simulink model "ARDC_IPMSM_Control"  (R2021b)
settings: Solver=VariableStepAuto  StartTime=0.0  StopTime=10  FixedStep=1e-6  MaxStep=1e-6  RelTol=1e-3
values from neighbouring files (symbols this model uses):
  B = 4.924e-4    (= 0.0004924)    [ARDC_PMSMControl_TreadmillLoad.m]
  J = 0.002700    (= 0.0027)    [ARDC_PMSMControl_TreadmillLoad.m]
  Kinv = Vdc/sqrt(2)    [ARDC_PMSMControl_TreadmillLoad.m]
  L_Stride = 1.8    [ARDC_PMSMControl_TreadmillLoad.m]
  Ld = 3.752e-4    (= 0.0003752)    [ARDC_PMSMControl_TreadmillLoad.m]
  Lq = 4.148e-4    (= 0.0004148)    [ARDC_PMSMControl_TreadmillLoad.m]
  P = 4    [ARDC_PMSMControl_TreadmillLoad.m]
  psim = 0.1194    [ARDC_PMSMControl_TreadmillLoad.m]
  R_roller = 0.1    [ARDC_PMSMControl_TreadmillLoad.m]
  Rs = 0.02    [ARDC_PMSMControl_TreadmillLoad.m]
  TreadMill_Enable = 1    [ARDC_PMSMControl_TreadmillLoad.m]
  Ts = 25e-6    (= 2.5e-05)    [ARDC_PMSMControl_TreadmillLoad.m]
  Tsw = 1/Fsw    (= 5e-05)    [ARDC_PMSMControl_TreadmillLoad.m]
  Vdc = 200    [ARDC_PMSMControl_TreadmillLoad.m]
undefined symbols (not defined in the file or in its folder): DiscIntNeverNeededParam
libraries: spsMosfetLib x6, slpidlib x3, spsVoltageMeasurementLib x3, simulink x2, spsPermanentMagnetSynchronousMachineLib x1, spsDCVoltageSourceLib x1, spsFirstOrderFilterLib x1, spspowerguiLib x1, spsTriangleGeneratorLib x1
settings Model: Creator=desai  LastModifiedBy=desai
settings DebuggingCC: UnderSpecifiedDimensionMsg=warning

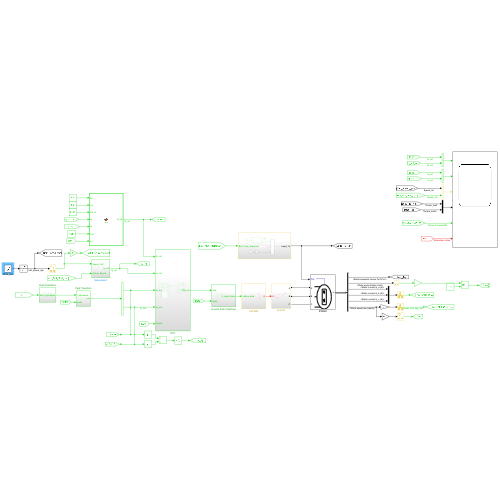
[thumbnail: Simulink's stored preview of the top-level diagram]
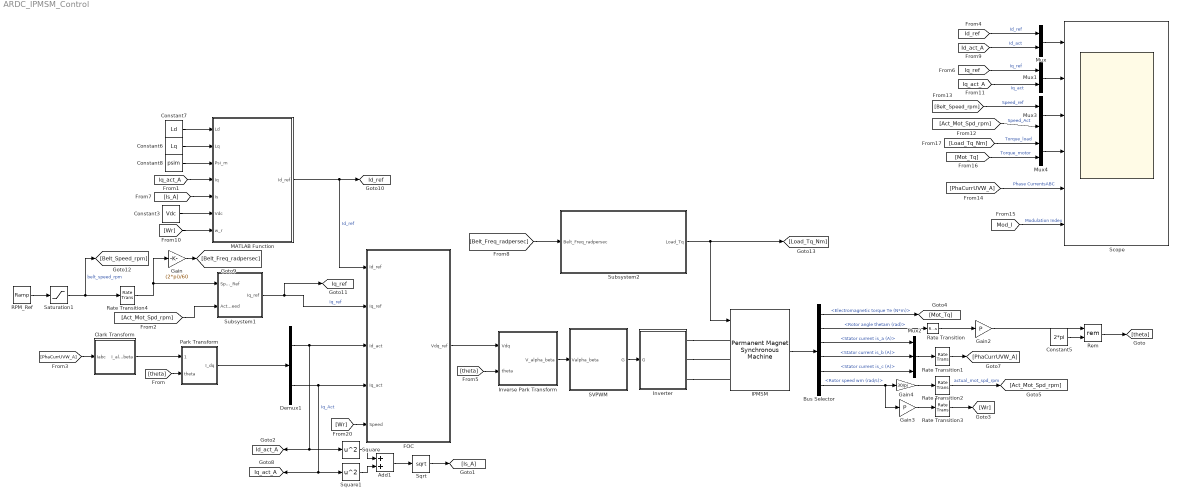
== system ARDC_IPMSM_Control ==
  Add1 : Sum
  Bus Selector : BusSelector  OutputSignals=Electromagnetic torque Te (N*m),Rotor angle thetam (rad),Stator current is_a (A),Stator current is_b (A),Stator current is_c (A),Rotor speed wm (rad/s)
  Clark Transform : Subsystem
  Constant3 : Constant  Value=Vdc  SampleTime=Ts
  Constant5 : Constant  Value=2*pi  SampleTime=Ts
  Constant6 : Constant  Value=Lq  SampleTime=Ts
  Constant7 : Constant  Value=Ld  SampleTime=Ts
  Constant8 : Constant  Value=psim  SampleTime=Ts
  Demux1 : Demux  Outputs=2
  FOC : Subsystem
  Gain : Gain  Gain=(2*pi)/60
  Gain2 : Gain  Gain=P
  Gain3 : Gain  Gain=P
  Gain4 : Gain  Gain=30/pi
  IPMSM : spsPermanentMagnetSynchronousMachineLib/Permanent Magnet Synchronous Machine  NbPhases=3  FluxDistribution=Sinusoidal  RotorType=Salient-pole  MechanicalLoad=Torque Tm  PresetModel=No  ShowDetailedParameters=on  MeasurementBus=off  Resistance=Rs  Inductance=8.5e-3  dqInductances=[Ld Lq]  La=0.000395  MachineConstant=Flux linkage established by magnets (V.s)  Flux=psim  VoltageCst=86.6271  TorqueCst=0.7164  Flat=120  Mechanical=[J B P 0]  PolePairs=P  InitialConditions=[0,0, 0,0]  InitialConditions5ph=[0 0 0 0 0 0]  RefAngle=Aligned with phase A axis (original Park)  IterativeDiscreteModel=Trapezoidal non iterative  TsBlock=-1  TsPowergui=0
  Inverse Park Transform : Subsystem
  Inverter : Subsystem
  MATLAB Function : MATLAB Function  TreatAsAtomicUnit=on
  Mux{,1,3..4} (4 alike) : Mux  Inputs=2
  Mux2 : Mux  Inputs=3
  Park Transform : Subsystem
  RPM_Ref : simulink/Sources/Ramp  slope=240  start=0  InitialOutput=0
  Rate Transition{,1..4} (5 alike) : RateTransition  OutPortSampleTime=Ts
  Rem : Math  Operator=rem  SaturateOnIntegerOverflow=on
  SVPWM : Subsystem
  Saturation1 : Saturate  UpperLimit=1200  LowerLimit=0
  Scope : Scope  NumInputPorts=6
  Sqrt : Sqrt  SaturateOnIntegerOverflow=on
  Square : Math  Operator=square  SaturateOnIntegerOverflow=on
  Square1 : Math  Operator=square  SaturateOnIntegerOverflow=on
  Subsystem1 : Subsystem
  Subsystem2 : Subsystem
  tag scope: Id_act_A=global, Id_ref=global, Iq_act_A=global, Iq_ref=global
  wires:
  IPMSM/1 -> Bus Selector/1
  Bus Selector/2 -> Rate Transition/1  "<Rotor angle thetam (rad)>"
  Mux2/1 -> Rate Transition1/1
  Clark Transform/1(I_alphabeta) -> Park Transform/1(I_alphabeta)
  SVPWM/1(G) -> Inverter/1(G)
  [Wr] -> FOC/5(Speed)
  FOC/1(Vdq_ref) -> Inverse Park Transform/1(Vdq)
  Demux1/2 -> [Iq_act_A], Square1/1, FOC/4(Iq_act)  "Iq_Act"
  Demux1/1 -> [Id_act_A], Square/1, FOC/3(Id_act)
  [theta] -> Inverse Park Transform/2(theta)
  Inverse Park Transform/1(V_alpha_beta) -> SVPWM/1(Valpha_beta)
  [theta] -> Park Transform/2(theta)
  Rate Transition/1 -> Gain2/1
  Constant5/1 -> Rem/2
  Rem/1 -> [theta]
  Gain3/1 -> Rate Transition3/1
  Bus Selector/1 -> [Mot_Tq]  "<Electromagnetic torque Te (N*m)>"
  [PhaCurrUVW_A] -> Clark Transform/1(Iabc)
  Gain4/1 -> Rate Transition2/1
  Add1/1 -> Sqrt/1
  Square/1 -> Add1/1
  Square1/1 -> Add1/2
  Sqrt/1 -> [Is_A]
  [Is_A] -> MATLAB Function/5(Is)
  [Iq_act_A] -> MATLAB Function/4(Iq)
  Constant3/1 -> MATLAB Function/6(Vdc)
  [Wr] -> MATLAB Function/7(w_r)
  Constant6/1 -> MATLAB Function/2(Lq)
  Constant7/1 -> MATLAB Function/1(Ld)
  Constant8/1 -> MATLAB Function/3(Psi_m)
  MATLAB Function/1(Id_ref) -> [Id_ref], FOC/1(Id_ref)  "Id_ref"
  RPM_Ref/1 -> Saturation1/1
  Saturation1/1 -> [Belt_Speed_rpm], Rate Transition4/1  "belt_speed_rpm"
  Rate Transition4/1 -> Gain/1, Subsystem1/1(Speed_Ref)
  [Act_Mot_Spd_rpm] -> Subsystem1/2(Actual_Speed)
  Gain/1 -> [Belt_Freq_radpersec]
  Bus Selector/3 -> Mux2/1  "<Stator current is_a (A)>"
  Bus Selector/4 -> Mux2/2  "<Stator current is_b (A)>"
  Bus Selector/5 -> Mux2/3  "<Stator current is_c (A)>"
  Bus Selector/6 -> Gain3/1, Gain4/1  "<Rotor speed wm (rad/s)>"
  Rate Transition3/1 -> [Wr]
  Gain2/1 -> Rem/1
  Subsystem1/1(Iq_ref) -> [Iq_ref], FOC/2(Iq_ref)  "Iq_ref"
  Rate Transition2/1 -> [Act_Mot_Spd_rpm]  "actual_mot_spd_rpm"
  Park Transform/1(I_dq) -> Demux1/1
  Rate Transition1/1 -> [PhaCurrUVW_A]
  [Id_ref] -> Mux/1  "Id_ref"
  [Id_act_A] -> Mux/2  "Id_act"
  [Iq_act_A] -> Mux1/2  "Iq_act"
  [Iq_ref] -> Mux1/1  "Iq_ref"
  [Belt_Speed_rpm] -> Mux3/1  "Speed_ref"
  [Act_Mot_Spd_rpm] -> Mux3/2  "Speed_Act"
  Mux/1 -> Scope/1
  Mux1/1 -> Scope/2
  Mux3/1 -> Scope/3
  [PhaCurrUVW_A] -> Scope/5  "Phase CurrentsABC"
  [Mod_I] -> Scope/6  "Modulation Index"
  [Mot_Tq] -> Mux4/2  "Torque_motor"
  [Load_Tq_Nm] -> Mux4/1  "Torque_load"
  Mux4/1 -> Scope/4
  [Belt_Freq_radpersec] -> Subsystem2/1(Belt_Freq_radpersec)
  Subsystem2/1(Load_Tq) -> IPMSM/1, [Load_Tq_Nm]
  connections:
  Inverter/RConn1 -- IPMSM/LConn1
  Inverter/RConn2 -- IPMSM/LConn2
  Inverter/RConn3 -- IPMSM/LConn3

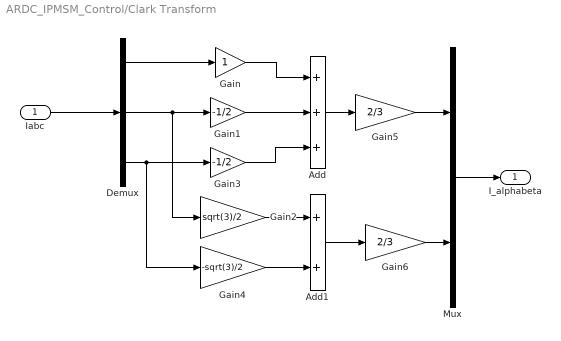
== system ARDC_IPMSM_Control/Clark Transform ==
  Iabc : Inport
  Add : Sum  Inputs=+++
  Add1 : Sum
  Demux : Demux  Outputs=3
  Gain : Gain
  Gain1 : Gain  Gain=-1/2
  Gain2 : Gain  Gain=sqrt(3)/2
  Gain3 : Gain  Gain=-1/2
  Gain4 : Gain  Gain=-sqrt(3)/2
  Gain5 : Gain  Gain=2/3
  Gain6 : Gain  Gain=2/3
  Mux : Mux  Inputs=2
  I_alphabeta : Outport  VectorParamsAs1DForOutWhenUnconnected=off
  wires:
  Gain/1 -> Add/1
  Demux/2 -> Gain1/1, Gain2/1
  Demux/3 -> Gain3/1, Gain4/1
  Gain1/1 -> Add/2
  Gain3/1 -> Add/3
  Gain4/1 -> Add1/2
  Gain2/1 -> Add1/1
  Demux/1 -> Gain/1
  Iabc/1 -> Demux/1
  Mux/1 -> I_alphabeta/1
  Add/1 -> Gain5/1
  Add1/1 -> Gain6/1
  Gain5/1 -> Mux/1
  Gain6/1 -> Mux/2

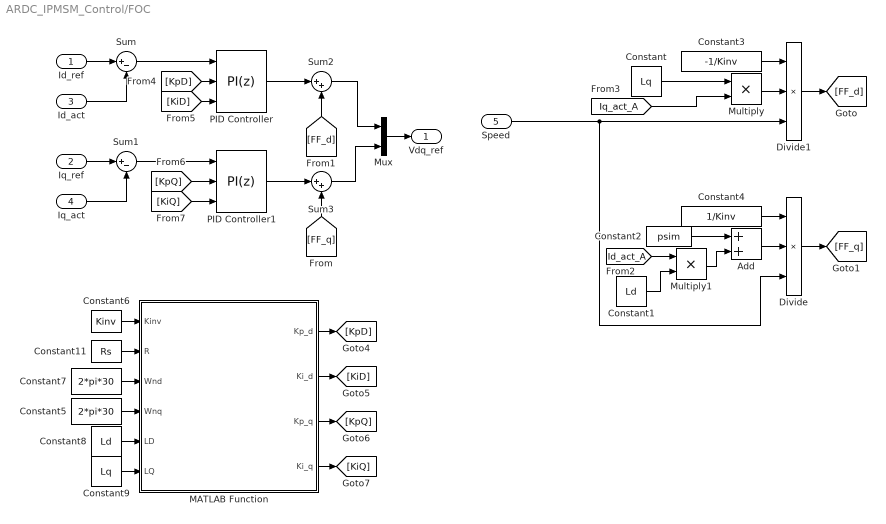
== system ARDC_IPMSM_Control/FOC ==
  Id_ref : Inport
  Iq_ref : Inport  Port=2
  Id_act : Inport  Port=3
  Iq_act : Inport  Port=4
  Speed : Inport  Port=5
  Add : Sum
  Constant : Constant  Value=Lq  SampleTime=Ts
  Constant1 : Constant  Value=Ld  SampleTime=Ts
  Constant11 : Constant  Value=Rs  SampleTime=Ts
  Constant2 : Constant  Value=psim  SampleTime=Ts
  Constant3 : Constant  Value=-1/Kinv  SampleTime=Ts
  Constant4 : Constant  Value=1/Kinv  SampleTime=Ts
  Constant5 : Constant  Value=2*pi*30  SampleTime=Ts
  Constant6 : Constant  Value=Kinv  SampleTime=Ts
  Constant7 : Constant  Value=2*pi*30  SampleTime=Ts
  Constant8 : Constant  Value=Ld  SampleTime=Ts
  Constant9 : Constant  Value=Lq  SampleTime=Ts
  Divide : Product  Inputs=***
  Divide1 : Product  Inputs=***
  MATLAB Function : MATLAB Function  TreatAsAtomicUnit=on
  Multiply : Product
  Multiply1 : Product
  Mux : Mux  Inputs=2
  PID Controller : slpidlib/PID Controller  Controller=PI  Form=Parallel  TimeDomain=Discrete-time  UseExternalTs=off  SampleTime=Ts  IntegratorMethod=Forward Euler  FilterMethod=Forward Euler  ControllerParametersSource=external  P=(2*1000*Ld - Rs)/Kinv  I=(Ld*2*1000*1000)/Kinv  D=0  UseFilter=on  N=100  TunerSelectOption=Transfer Function Based (PID Tuner App)  InitialConditionSource=internal  InitialConditionForIntegrator=0  InitialConditionForFilter=0  DifferentiatorICPrevScaledInput=0  ExternalReset=none  IgnoreLimit=on  TrackingMode=off  Kt=1  LimitOutput=off  SatLimitsSource=internal  UpperSaturationLimit=inf  LowerSaturationLimit=-inf  LinearizeAsGain=on  AntiWindupMode=none  Kb=1  POutMin=[]  POutMax=[]  IOutMin=[]  IOutMax=[]  DOutMin=[]  DOutMax=[]  NOutMin=[]  NOutMax=[]  SumOutMin=[]  SumOutMax=[]  SaturationOutMin=[]  SaturationOutMax=[]  PParamMin=[]  PParamMax=[]  IParamMin=[]  IParamMax=[]  DParamMin=[]  DParamMax=[]  NParamMin=[]  NParamMax=[]  KbParamMin=[]  KbParamMax=[]  KtParamMin=[]  KtParamMax=[]  KbOutMin=[]  KbOutMax=[]  KtOutMin=[]  KtOutMax=[]  IntegratorOutMin=[]  IntegratorOutMax=[]  FilterOutMin=[]  FilterOutMax=[]  SumI1OutMin=[]  SumI1OutMax=[]  SumI2OutMin=[]  SumI2OutMax=[]  SumI3OutMin=[]  SumI3OutMax=[]  SumI4OutMin=[]  SumI4OutMax=[]  SumDOutMin=[]  SumDOutMax=[]  DifferentiatorOutMin=[]  DifferentiatorOutMax=[]  FilterDiffOutCoefMin=[]  FilterDiffOutCoefMax=[]  ReciprocalOutMin=[]  ReciprocalOutMax=[]  SumDenOutMin=[]  SumDenOutMax=[]  SumNumOutMin=[]  SumNumOutMax=[]  DivideOutMin=[]  DivideOutMax=[]  UdiffTsProdOutMin=[]  UdiffTsProdOutMax=[]  NTsProdOutMin=[]  NTsProdOutMax=[]  UintegralTsProdOutMin=[]  UintegralTsProdOutMax=[]  UngainTsProdOutMin=[]  UngainTsProdOutMax=[]  IntegratorContinuousStateAttributes=''  IntegratorStateMustResolveToSignalObject=off  IntegratorRTWStateStorageClass=Auto  FilterContinuousStateAttributes=''  FilterStateMustResolveToSignalObject=off  FilterRTWStateStorageClass=Auto  ParallelPVariant=ExternalParameters  IdealPVariant=Disabled  IVariant=ExternalParameters  DVariant=Disabled  IntegratorVariant=Discrete  SatVariant=Disabled  AWVariant=Passthrough  PCopyVariant=Disabled  TRVariant=Disabled  FdbkBlocksVariant=Forward  IdealPFdbkVariant=Disabled  SatFdbkVariant=Disabled  DerivativeFilterVariant=Disabled  NVariant=Disabled  NCopyVariant=Disabled_SignalSpec  FilterICVariant=Disabled  IntegratorICVariant=InternalICs  ExternalResetVariant=Disabled  TRSumVariant=Passthrough  SumFdbkVariant=Disabled  SumVariant=Sum_PI  TsampFilterVariant=InternalTs  TsampNgainVariant=Passthrough  TsampIntegralVariant=Passthrough  ExternalSaturationOutDataTypeStr=Inherit: Same as second input
  PID Controller1 : slpidlib/PID Controller  Controller=PI  Form=Parallel  TimeDomain=Discrete-time  UseExternalTs=off  SampleTime=Ts  IntegratorMethod=Forward Euler  FilterMethod=Forward Euler  ControllerParametersSource=external  P=(2*1000*Lq - Rs)/Kinv  I=(Lq*2*1000*1000)/Kinv  D=0  UseFilter=on  N=100  TunerSelectOption=Transfer Function Based (PID Tuner App)  InitialConditionSource=internal  InitialConditionForIntegrator=0  InitialConditionForFilter=0  DifferentiatorICPrevScaledInput=0  ExternalReset=none  TrackingMode=off  Kt=1  LimitOutput=off  SatLimitsSource=internal  UpperSaturationLimit=inf  LowerSaturationLimit=-inf  LinearizeAsGain=on  AntiWindupMode=none  Kb=1  POutMin=[]  POutMax=[]  IOutMin=[]  IOutMax=[]  DOutMin=[]  DOutMax=[]  NOutMin=[]  NOutMax=[]  SumOutMin=[]  SumOutMax=[]  SaturationOutMin=[]  SaturationOutMax=[]  PParamMin=[]  PParamMax=[]  IParamMin=[]  IParamMax=[]  DParamMin=[]  DParamMax=[]  NParamMin=[]  NParamMax=[]  KbParamMin=[]  KbParamMax=[]  KtParamMin=[]  KtParamMax=[]  KbOutMin=[]  KbOutMax=[]  KtOutMin=[]  KtOutMax=[]  IntegratorOutMin=[]  IntegratorOutMax=[]  FilterOutMin=[]  FilterOutMax=[]  SumI1OutMin=[]  SumI1OutMax=[]  SumI2OutMin=[]  SumI2OutMax=[]  SumI3OutMin=[]  SumI3OutMax=[]  SumI4OutMin=[]  SumI4OutMax=[]  SumDOutMin=[]  SumDOutMax=[]  DifferentiatorOutMin=[]  DifferentiatorOutMax=[]  FilterDiffOutCoefMin=[]  FilterDiffOutCoefMax=[]  ReciprocalOutMin=[]  ReciprocalOutMax=[]  SumDenOutMin=[]  SumDenOutMax=[]  SumNumOutMin=[]  SumNumOutMax=[]  DivideOutMin=[]  DivideOutMax=[]  UdiffTsProdOutMin=[]  UdiffTsProdOutMax=[]  NTsProdOutMin=[]  NTsProdOutMax=[]  UintegralTsProdOutMin=[]  UintegralTsProdOutMax=[]  UngainTsProdOutMin=[]  UngainTsProdOutMax=[]  IntegratorContinuousStateAttributes=''  IntegratorStateMustResolveToSignalObject=off  IntegratorRTWStateStorageClass=Auto  FilterContinuousStateAttributes=''  FilterStateMustResolveToSignalObject=off  FilterRTWStateStorageClass=Auto  ParallelPVariant=ExternalParameters  IdealPVariant=Disabled  IVariant=ExternalParameters  DVariant=Disabled  IntegratorVariant=Discrete  SatVariant=Disabled  AWVariant=Passthrough  PCopyVariant=Disabled  TRVariant=Disabled  FdbkBlocksVariant=Forward  IdealPFdbkVariant=Disabled  SatFdbkVariant=Disabled  DerivativeFilterVariant=Disabled  NVariant=Disabled  NCopyVariant=Disabled_SignalSpec  FilterICVariant=Disabled  IntegratorICVariant=InternalICs  ExternalResetVariant=Disabled  TRSumVariant=Passthrough  SumFdbkVariant=Disabled  SumVariant=Sum_PI  TsampFilterVariant=InternalTs  TsampNgainVariant=Passthrough  TsampIntegralVariant=Passthrough  ExternalSaturationOutDataTypeStr=Inherit: Same as second input
  Sum : Sum  Inputs=|+-
  Sum1 : Sum  Inputs=|+-
  Sum2 : Sum  Inputs=|++
  Sum3 : Sum  Inputs=|++
  Vdq_ref : Outport  VectorParamsAs1DForOutWhenUnconnected=off
  wires:
  Id_ref/1 -> Sum/1
  Iq_ref/1 -> Sum1/1
  Id_act/1 -> Sum/2
  Sum1/1 -> PID Controller1/1
  Sum/1 -> PID Controller/1
  PID Controller/1 -> Sum2/1
  PID Controller1/1 -> Sum3/1
  Sum2/1 -> Mux/1
  Sum3/1 -> Mux/2
  Mux/1 -> Vdq_ref/1
  Iq_act/1 -> Sum1/2
  Constant1/1 -> Multiply1/2
  Constant/1 -> Multiply/1
  Multiply/1 -> Divide1/2
  [FF_q] -> Sum3/2
  [FF_d] -> Sum2/2
  Divide/1 -> [FF_q]
  Speed/1 -> Divide/3, Divide1/3
  Multiply1/1 -> Add/2
  Constant2/1 -> Add/1
  Add/1 -> Divide/2
  [Id_act_A] -> Multiply1/1
  [Iq_act_A] -> Multiply/2
  Constant3/1 -> Divide1/1
  Divide1/1 -> [FF_d]
  Constant4/1 -> Divide/1
  Constant8/1 -> MATLAB Function/5(LD)
  Constant9/1 -> MATLAB Function/6(LQ)
  Constant7/1 -> MATLAB Function/3(Wnd)
  MATLAB Function/4(Ki_q) -> [KiQ]
  MATLAB Function/3(Kp_q) -> [KpQ]
  MATLAB Function/2(Ki_d) -> [KiD]
  MATLAB Function/1(Kp_d) -> [KpD]
  [KpD] -> PID Controller/2
  [KiD] -> PID Controller/3
  [KpQ] -> PID Controller1/2
  [KiQ] -> PID Controller1/3
  Constant6/1 -> MATLAB Function/1(Kinv)
  Constant11/1 -> MATLAB Function/2(R)
  Constant5/1 -> MATLAB Function/4(Wnq)

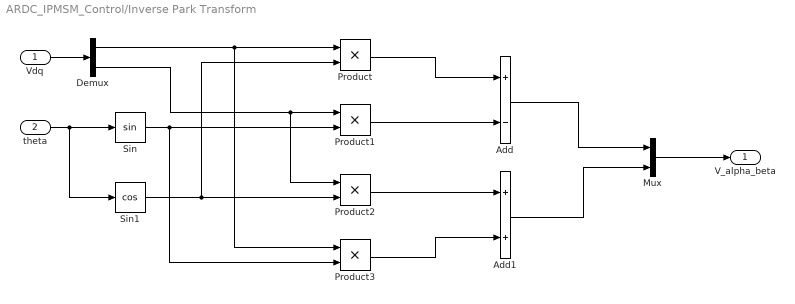
== system ARDC_IPMSM_Control/Inverse Park Transform ==
  Vdq : Inport
  theta : Inport  Port=2
  Add : Sum  Inputs=+-
  Add1 : Sum
  Demux : Demux  Outputs=2
  Mux : Mux  Inputs=2
  Product{,1..3} (4 alike) : Product
  Sin : Trigonometry
  Sin1 : Trigonometry  Operator=cos
  V_alpha_beta : Outport  VectorParamsAs1DForOutWhenUnconnected=off
  wires:
  Vdq/1 -> Demux/1
  Demux/1 -> Product/1, Product3/1
  Sin1/1 -> Product2/2, Product/2
  Product/1 -> Add/1
  Demux/2 -> Product2/1, Product1/1
  Product1/1 -> Add/2
  Sin/1 -> Product1/2, Product3/2
  Product3/1 -> Add1/2
  Product2/1 -> Add1/1
  theta/1 -> Sin/1, Sin1/1
  Add/1 -> Mux/1
  Add1/1 -> Mux/2
  Mux/1 -> V_alpha_beta/1

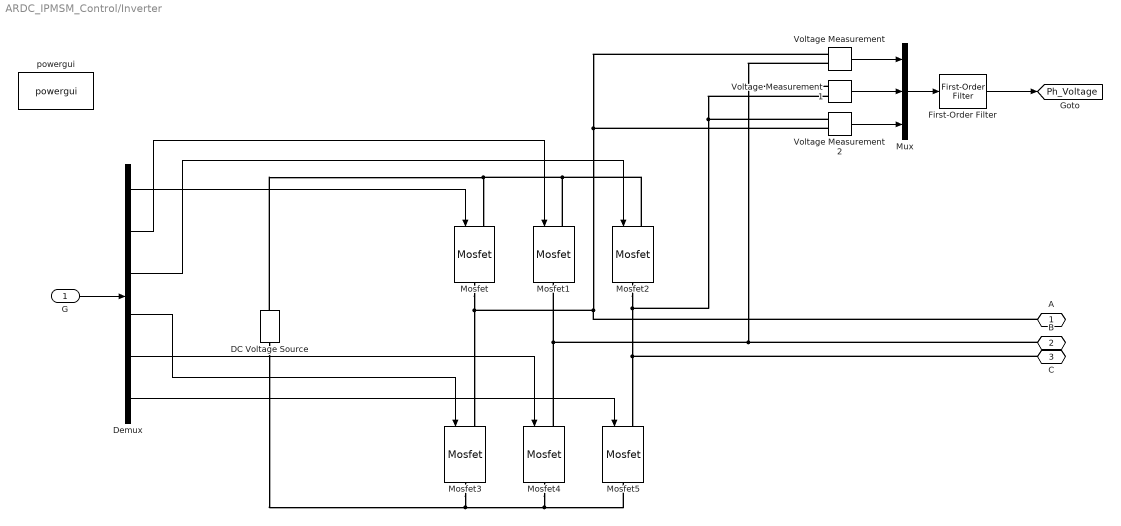
== system ARDC_IPMSM_Control/Inverter ==
  G : Inport
  DC Voltage Source : spsDCVoltageSourceLib/DC Voltage Source  Amplitude=Vdc  Measurements=None
  Demux : Demux  Outputs=6
  First-Order Filter : spsFirstOrderFilterLib/First-Order Filter  FilterType=Lowpass  Tc=1/(2*pi*200)  Ts=0  Initialize=off  Vac_Init=[0, 0, 60]  Vdc_Init=0  PlotResponse=off  FreqRange="[0,  200,  1]"
  Mosfet{,1..5} (6 alike) : spsMosfetLib/Mosfet  Ron=0.05  Lon=0  Rd=0.01  Vfd=0  IC=0  Rs=1e5  Cs=inf  Measurements=off
  Mux : Mux  Inputs=3
  Voltage Measurement : spsVoltageMeasurementLib/Voltage Measurement  PhasorSimulation=off  OutputType=Complex  PSBequivalent=0
  Voltage Measurement1 : spsVoltageMeasurementLib/Voltage Measurement  PhasorSimulation=off  OutputType=Complex  PSBequivalent=0
  Voltage Measurement2 : spsVoltageMeasurementLib/Voltage Measurement  PhasorSimulation=off  OutputType=Complex  PSBequivalent=0
  powergui : spspowerguiLib/powergui  Priority=1  SimulationMode=Continuous  SampleTime=50e-6  frequency=60  Iterations=50  frequencyindice=0  Pbase=100e6  ErrMax=1e-4  UnitsV=kV  UnitsW=MW  buscounter=0  FunctionMessages=off  echomessages=off  EnableUseOfTLC=off  CurrentSourceSwitches=off  DisableSnubberDevices=off  DisableRonSwitches=off  DisableVfSwitches=off  DisplayEquations=off  AutomaticDiscreteSolvers=off  SolverType=Tustin/Backward Euler (TBE)  Interpol=off  ExternalGateDelay=off  methode=off  Ts=100  x0status=blocks  SPID=on  SwTol=0  HookPort=off  NonlinearTolerance=1e-4  nMaxIteration=100  ContinueOnMaxIteration=off  RestoreLinks=warning  ResistiveCurrentMeasurement=off  Frange=[0:2:500]  Ylog=off  Xlog=on  ShowGrid=off  save=off  variable=ZData  structure=0  ZoomFFT=off  StartTime=0.0  cycles=1  DisplayStyle=1  fundamental=60  FreqAxis=off  MaxFrequency=1000  frequencyindicesteady=1  RmsSteady=1  display=off
  A : PMIOPort  Side=Right
  B : PMIOPort  Port=2  Side=Right
  C : PMIOPort  Port=3  Side=Right
  tag scope: Ph_Voltage=global
  wires:
  G/1 -> Demux/1
  Demux/1 -> Mosfet/1
  Demux/2 -> Mosfet1/1
  Demux/3 -> Mosfet2/1
  Demux/4 -> Mosfet3/1
  Demux/5 -> Mosfet4/1
  Demux/6 -> Mosfet5/1
  Voltage Measurement/1 -> Mux/1
  Voltage Measurement1/1 -> Mux/2
  Voltage Measurement2/1 -> Mux/3
  Mux/1 -> First-Order Filter/1
  First-Order Filter/1 -> [Ph_Voltage]
  connections:
  Mosfet2/LConn1 -- DC Voltage Source/RConn1 -- Mosfet/LConn1 -- Mosfet1/LConn1
  Mosfet3/RConn1 -- Mosfet5/RConn1 -- Mosfet4/RConn1 -- DC Voltage Source/LConn1
  Mosfet2/RConn1 -- Voltage Measurement2/LConn1 -- Voltage Measurement1/LConn2 -- Mosfet5/LConn1 -- C/RConn1
  Mosfet/RConn1 -- A/RConn1 -- Voltage Measurement2/LConn2 -- Voltage Measurement/LConn1 -- Mosfet3/LConn1
  B/RConn1 -- Mosfet1/RConn1 -- Mosfet4/LConn1 -- Voltage Measurement1/LConn1 -- Voltage Measurement/LConn2

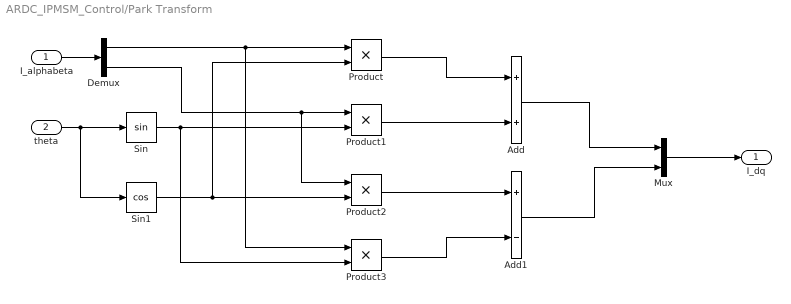
== system ARDC_IPMSM_Control/Park Transform ==
  I_alphabeta : Inport
  theta : Inport  Port=2
  Add : Sum
  Add1 : Sum  Inputs=+-
  Demux : Demux  Outputs=2
  Mux : Mux  Inputs=2
  Product{,1..3} (4 alike) : Product
  Sin : Trigonometry
  Sin1 : Trigonometry  Operator=cos
  I_dq : Outport  VectorParamsAs1DForOutWhenUnconnected=off
  wires:
  Mux/1 -> I_dq/1
  Add1/1 -> Mux/2
  Add/1 -> Mux/1
  theta/1 -> Sin1/1, Sin/1
  Product2/1 -> Add1/1
  Product3/1 -> Add1/2
  Sin/1 -> Product3/2, Product1/2
  Product1/1 -> Add/2
  Demux/2 -> Product1/1, Product2/1
  Product/1 -> Add/1
  Sin1/1 -> Product/2, Product2/2
  Demux/1 -> Product3/1, Product/1
  I_alphabeta/1 -> Demux/1

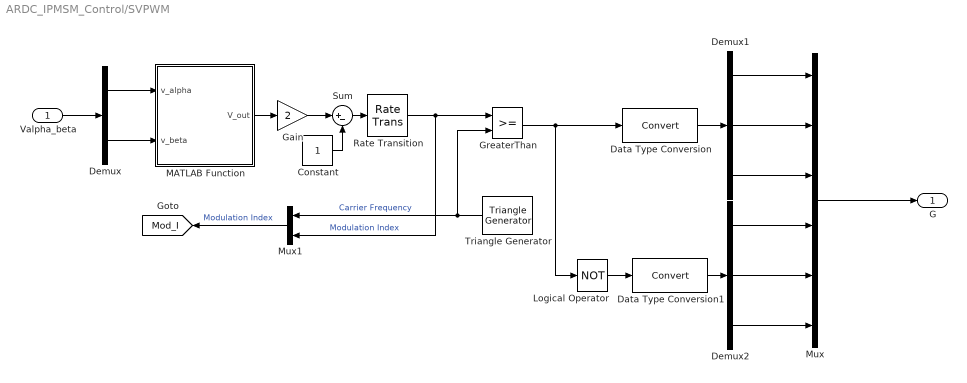
== system ARDC_IPMSM_Control/SVPWM ==
  Valpha_beta : Inport
  Constant : Constant
  Data Type Conversion : DataTypeConversion
  Data Type Conversion1 : DataTypeConversion
  Demux : Demux  Outputs=2
  Demux1 : Demux  Outputs=3
  Demux2 : Demux  Outputs=3
  Gain : Gain  Gain=2
  GreaterThan : RelationalOperator  OutDataTypeStr=boolean  RndMeth=Simplest
  Logical Operator : Logic  Operator=NOT  AllPortsSameDT=off  OutDataTypeStr=boolean
  MATLAB Function : MATLAB Function  TreatAsAtomicUnit=on
  Mux : Mux  Inputs=6
  Mux1 : Mux  Inputs=2
  Rate Transition : RateTransition  OutPortSampleTime=Tsw/40
  Sum : Sum  Inputs=|+-
  Triangle Generator : spsTriangleGeneratorLib/Triangle Generator  Freq=Fsw  Phase=0  Ts=Tsw/40
  G : Outport  VectorParamsAs1DForOutWhenUnconnected=off
  tag scope: Mod_I=global
  wires:
  MATLAB Function/1(V_out) -> Gain/1
  Valpha_beta/1 -> Demux/1
  Demux/1 -> MATLAB Function/1(v_alpha)
  Demux/2 -> MATLAB Function/2(v_beta)
  GreaterThan/1 -> Logical Operator/1, Data Type Conversion/1
  Logical Operator/1 -> Data Type Conversion1/1
  Triangle Generator/1 -> GreaterThan/2, Mux1/1  "Carrier Frequency"
  Mux/1 -> G/1
  Data Type Conversion/1 -> Demux1/1
  Demux1/3 -> Mux/3
  Demux1/2 -> Mux/2
  Demux1/1 -> Mux/1
  Demux2/1 -> Mux/4
  Demux2/2 -> Mux/5
  Demux2/3 -> Mux/6
  Data Type Conversion1/1 -> Demux2/1
  Rate Transition/1 -> GreaterThan/1, Mux1/2  "Modulation Index"
  Mux1/1 -> [Mod_I]  "Modulation Index"
  Gain/1 -> Sum/1
  Sum/1 -> Rate Transition/1
  Constant/1 -> Sum/2

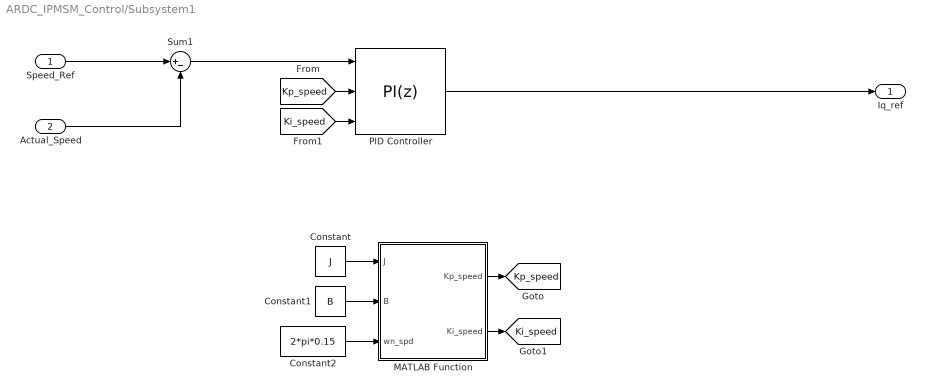
== system ARDC_IPMSM_Control/Subsystem1 ==
  Speed_Ref : Inport
  Actual_Speed : Inport  Port=2
  Constant : Constant  Value=J  SampleTime=Ts
  Constant1 : Constant  Value=B  SampleTime=Ts
  Constant2 : Constant  Value=2*pi*0.15  SampleTime=Ts
  MATLAB Function : MATLAB Function  TreatAsAtomicUnit=on
  PID Controller : slpidlib/PID Controller  Controller=PI  Form=Parallel  TimeDomain=Discrete-time  UseExternalTs=off  SampleTime=Ts  IntegratorMethod=Forward Euler  FilterMethod=Forward Euler  ControllerParametersSource=external  P=1  I=1  D=0  UseFilter=on  N=100  TunerSelectOption=Transfer Function Based (PID Tuner App)  InitialConditionSource=internal  InitialConditionForIntegrator=0  InitialConditionForFilter=0  DifferentiatorICPrevScaledInput=0  ExternalReset=none  TrackingMode=off  Kt=1  LimitOutput=off  SatLimitsSource=internal  UpperSaturationLimit=inf  LowerSaturationLimit=-inf  LinearizeAsGain=on  AntiWindupMode=none  Kb=1  POutMin=[]  POutMax=[]  IOutMin=[]  IOutMax=[]  DOutMin=[]  DOutMax=[]  NOutMin=[]  NOutMax=[]  SumOutMin=[]  SumOutMax=[]  SaturationOutMin=[]  SaturationOutMax=[]  PParamMin=[]  PParamMax=[]  IParamMin=[]  IParamMax=[]  DParamMin=[]  DParamMax=[]  NParamMin=[]  NParamMax=[]  KbParamMin=[]  KbParamMax=[]  KtParamMin=[]  KtParamMax=[]  KbOutMin=[]  KbOutMax=[]  KtOutMin=[]  KtOutMax=[]  IntegratorOutMin=[]  IntegratorOutMax=[]  FilterOutMin=[]  FilterOutMax=[]  SumI1OutMin=[]  SumI1OutMax=[]  SumI2OutMin=[]  SumI2OutMax=[]  SumI3OutMin=[]  SumI3OutMax=[]  SumI4OutMin=[]  SumI4OutMax=[]  SumDOutMin=[]  SumDOutMax=[]  DifferentiatorOutMin=[]  DifferentiatorOutMax=[]  FilterDiffOutCoefMin=[]  FilterDiffOutCoefMax=[]  ReciprocalOutMin=[]  ReciprocalOutMax=[]  SumDenOutMin=[]  SumDenOutMax=[]  SumNumOutMin=[]  SumNumOutMax=[]  DivideOutMin=[]  DivideOutMax=[]  UdiffTsProdOutMin=[]  UdiffTsProdOutMax=[]  NTsProdOutMin=[]  NTsProdOutMax=[]  UintegralTsProdOutMin=[]  UintegralTsProdOutMax=[]  UngainTsProdOutMin=[]  UngainTsProdOutMax=[]  IntegratorContinuousStateAttributes=''  IntegratorStateMustResolveToSignalObject=off  IntegratorRTWStateStorageClass=Auto  FilterContinuousStateAttributes=''  FilterStateMustResolveToSignalObject=off  FilterRTWStateStorageClass=Auto  ParallelPVariant=ExternalParameters  IdealPVariant=Disabled  IVariant=ExternalParameters  DVariant=Disabled  IntegratorVariant=Discrete  SatVariant=Disabled  AWVariant=Passthrough  PCopyVariant=Disabled  TRVariant=Disabled  FdbkBlocksVariant=Forward  IdealPFdbkVariant=Disabled  SatFdbkVariant=Disabled  DerivativeFilterVariant=Disabled  NVariant=Disabled  NCopyVariant=Disabled_SignalSpec  FilterICVariant=Disabled  IntegratorICVariant=InternalICs  ExternalResetVariant=Disabled  TRSumVariant=Passthrough  SumFdbkVariant=Disabled  SumVariant=Sum_PI  TsampFilterVariant=InternalTs  TsampNgainVariant=Passthrough  TsampIntegralVariant=Passthrough  ExternalSaturationOutDataTypeStr=Inherit: Same as second input
  Sum1 : Sum  Inputs=|+-
  Iq_ref : Outport
  tag scope: Ki_speed=global, Kp_speed=global
  wires:
  [Kp_speed] -> PID Controller/2
  [Ki_speed] -> PID Controller/3
  MATLAB Function/1(Kp_speed) -> [Kp_speed]
  MATLAB Function/2(Ki_speed) -> [Ki_speed]
  Constant/1 -> MATLAB Function/1(J)
  Constant1/1 -> MATLAB Function/2(B)
  Constant2/1 -> MATLAB Function/3(wn_spd)
  Sum1/1 -> PID Controller/1
  Speed_Ref/1 -> Sum1/1
  Actual_Speed/1 -> Sum1/2
  PID Controller/1 -> Iq_ref/1

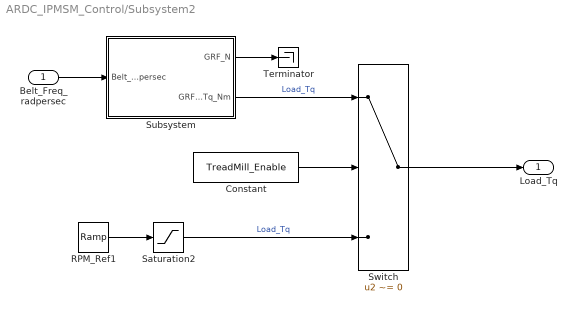
== system ARDC_IPMSM_Control/Subsystem2 ==
  Belt_Freq_radpersec : Inport
  Constant : Constant  Value=TreadMill_Enable
  RPM_Ref1 : simulink/Sources/Ramp  slope=100  start=0  InitialOutput=0
  Saturation2 : Saturate  UpperLimit=5  LowerLimit=0
  Subsystem : Subsystem
  Switch : Switch  Criteria=u2 ~= 0
  Terminator : Terminator
  Load_Tq : Outport
  wires:
  Subsystem/1(GRF_N) -> Terminator/1
  Belt_Freq_radpersec/1 -> Subsystem/1(Belt_Freq_radpersec)
  RPM_Ref1/1 -> Saturation2/1
  Saturation2/1 -> Switch/3  "Load_Tq"
  Switch/1 -> Load_Tq/1
  Subsystem/2(GRF_LoadTq_Nm) -> Switch/1  "Load_Tq"
  Constant/1 -> Switch/2

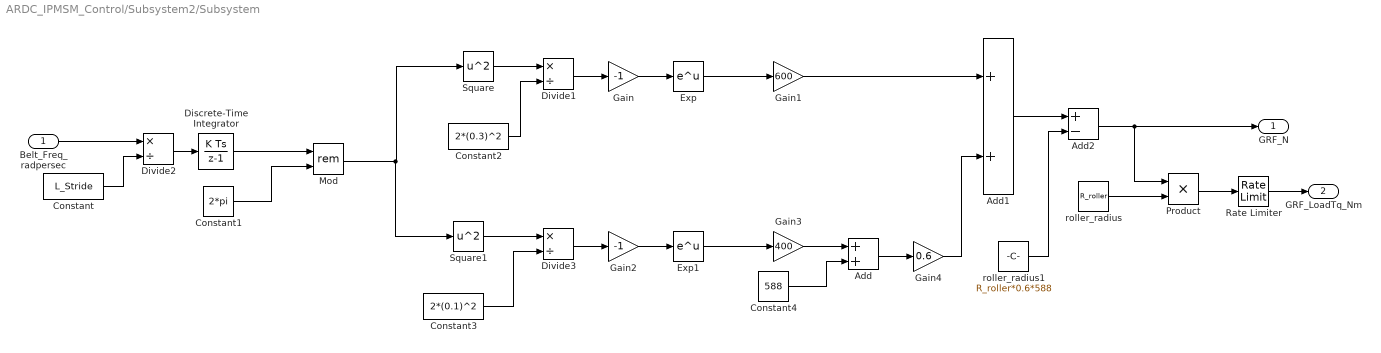
== system ARDC_IPMSM_Control/Subsystem2/Subsystem ==
  Belt_Freq_radpersec : Inport
  Add : Sum
  Add1 : Sum
  Add2 : Sum  Inputs=+-
  Constant : Constant  Value=L_Stride  SampleTime=Ts
  Constant1 : Constant  Value=2*pi  SampleTime=Ts
  Constant2 : Constant  Value=2*(0.3)^2  SampleTime=Ts
  Constant3 : Constant  Value=2*(0.1)^2  SampleTime=Ts
  Constant4 : Constant  Value=588  SampleTime=Ts
  Discrete-Time Integrator : DiscreteIntegrator  SampleTime=-1  ICPrevOutput=DiscIntNeverNeededParam  ICPrevScaledInput=DiscIntNeverNeededParam
  Divide1 : Product  Inputs=*/
  Divide2 : Product  Inputs=*/
  Divide3 : Product  Inputs=*/
  Exp : Math  SaturateOnIntegerOverflow=on
  Exp1 : Math  SaturateOnIntegerOverflow=on
  Gain : Gain  Gain=-1
  Gain1 : Gain  Gain=600
  Gain2 : Gain  Gain=-1
  Gain3 : Gain  Gain=400
  Gain4 : Gain  Gain=0.6
  Mod : Math  Operator=rem  SaturateOnIntegerOverflow=on
  Product : Product
  Rate Limiter : RateLimiter  RisingSlewLimit=500  FallingSlewLimit=-500  SampleTimeMode=inherited
  Square : Math  Operator=square  SaturateOnIntegerOverflow=on
  Square1 : Math  Operator=square  SaturateOnIntegerOverflow=on
  roller_radius : Constant  Value=R_roller  SampleTime=Ts
  roller_radius1 : Constant  Value=R_roller*0.6*588  SampleTime=Ts
  GRF_N : Outport
  GRF_LoadTq_Nm : Outport  Port=2
  wires:
  Constant1/1 -> Mod/2
  Discrete-Time Integrator/1 -> Mod/1
  roller_radius/1 -> Product/2
  Belt_Freq_radpersec/1 -> Divide2/1
  Divide2/1 -> Discrete-Time Integrator/1
  Constant/1 -> Divide2/2
  Constant2/1 -> Divide1/2
  Square/1 -> Divide1/1
  Divide1/1 -> Gain/1
  Gain/1 -> Exp/1
  Exp/1 -> Gain1/1
  Gain1/1 -> Add1/1
  Gain3/1 -> Add/1
  Exp1/1 -> Gain3/1
  Gain2/1 -> Exp1/1
  Divide3/1 -> Gain2/1
  Square1/1 -> Divide3/1
  Constant3/1 -> Divide3/2
  Constant4/1 -> Add/2
  Add/1 -> Gain4/1
  Gain4/1 -> Add1/2
  roller_radius1/1 -> Add2/2
  Add1/1 -> Add2/1
  Add2/1 -> Product/1, GRF_N/1
  Mod/1 -> Square1/1, Square/1
  Product/1 -> Rate Limiter/1
  Rate Limiter/1 -> GRF_LoadTq_Nm/1

== matlab function ARDC_IPMSM_Control/FOC/MATLAB Function ==
  data: Kinv input; Kp_d output; R input; Wnd input; Wnq input; LD input; LQ input; Ki_d output; Kp_q output; Ki_q output
function [Kp_d, Ki_d, Kp_q, Ki_q] = fcn(Kinv,R,Wnd,Wnq,LD,LQ)
zeta = 1/sqrt(2);
Ke = Kinv;

Te_d = LD/R;
Te_q = LQ/R;


Kp_d = (2*zeta*Wnd*Te_d - 1)/Ke;
Kp_q = (2*zeta*Wnq*Te_q - 1)/Ke;

Ki_d = Wnd^2*Te_d/Ke;  
Ki_q = Wnq^2*Te_q/Ke;
end

== matlab function ARDC_IPMSM_Control/SVPWM/MATLAB Function ==
  data: v_alpha input; V_out output; v_beta input
function V_out= fcn(v_alpha,v_beta)
vref=sqrt(v_alpha^2+v_beta^2);
angle=atan2d(v_beta,v_alpha);
%del_V = (sqrt(3)/2)-vref;
if vref> 1
    vref=1;
end
%% Initialize variables

sector=0;
va=0;
vb=0;
vc=0;
ang=0;

if(angle>=0 && angle<60)	    %condition for sector one
    sector=1;
    ang=angle*pi/180;
end
if(angle>=60 && angle<120)	    %condition for sector two
	ang=angle*pi/180-pi/3;
    sector=2;
end
if(angle>=120 && angle<=180)	%condition for sector three
	ang=angle*pi/180-2*pi/3;
    sector=3;
end
if(angle>=-180 && angle<-120)	%condition for sector four
	ang=angle*pi/180-3*pi/3;
    sector=4;
end
if(angle>=-120 && angle<-60)	%condition for sector five
	ang=angle*pi/180-4*pi/3;
    sector=5;
end
if(angle>=-60 && angle<0)	    %condition for sector six
	ang=angle*pi/180-5*pi/3;
    sector=6;   
end

ta= (vref)*(sqrt(3)/2)*(sin(pi/3-ang)/sin(pi/3));
tb= (vref)*(sqrt(3)/2)*(sin(ang))/(sin(pi/3));
t0=1-ta-tb;

m1=ta+tb+(t0)/2;
m0=(t0)/2;
ma=ta+(t0)/2;
mb=tb+(t0)/2;

switch sector
    case 1
        va=m1;
        vb=mb;
        vc=m0;
    case 2
        va=ma;
        vb=m1;
        vc=m0;
    case 3
        va=m0;
        vb=m1;
        vc=mb;
    case 4
        va=m0;
        vb=ma;
        vc=m1;
    case 5
        va=mb;
        vb=m0;
        vc=m1;
    case 6
        va=m1;
        vb=m0;
        vc=ma;
end    
V_out = [va;vb;vc];

== matlab function ARDC_IPMSM_Control/MATLAB Function ==
  data: Id_ref output; Ld input; Lq input; Psi_m input; Iq input; Is input; Vdc input; w_r input
function Id_ref  = fcn(Ld,Lq,Psi_m,Iq,Is,Vdc,w_r)
Vsmax = 0.9*(Vdc/sqrt(2));
Psi_max = Vsmax/w_r;
%Id Reference Generation 
Id_mtpa = (-Psi_m + sqrt(Psi_m^2 + 8*((Ld-Lq)*Is)^2))/(4*(Ld-Lq));
Psi_q = Lq*Iq;
Psi_d_sqr = Psi_max^2 - Psi_q^2;
if Psi_d_sqr < 0
    Id_FW = -Psi_m/Ld;
else
    Id_FW = (sqrt(Psi_d_sqr) - Psi_m)/Ld;
end
%Iq Reference Generation 
if Id_FW > Id_mtpa
    Id_ref = Id_mtpa;
else
    Id_ref = Id_FW;
end

end

== matlab function ARDC_IPMSM_Control/Subsystem1/MATLAB Function ==
  data: J input; Kp_speed output; B input; wn_spd input; Ki_speed output
function [Kp_speed, Ki_speed] = fcn(J,B,wn_spd)
%% Speed Control Loop Coefficients
zeta = 1/sqrt(2);
Tspd = J/B;

Kp_speed = (2*zeta*wn_spd*Tspd -1);
Ki_speed = (Tspd*wn_spd^2); 

end
